simulink model "model_3"  (R2023b)
settings: Solver=VariableStepAuto  StartTime=0.0  StopTime=10  RelTol=1e-3
values from neighbouring files (symbols this model uses):
  k = acker(A, B, [s_b s_b s_b])    [obiekt.m]
settings Model: Creator=pavig  LastModifiedBy=pavig

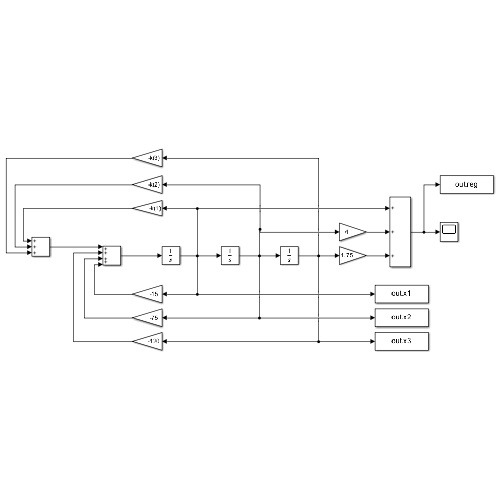
[thumbnail: Simulink's stored preview of the top-level diagram]
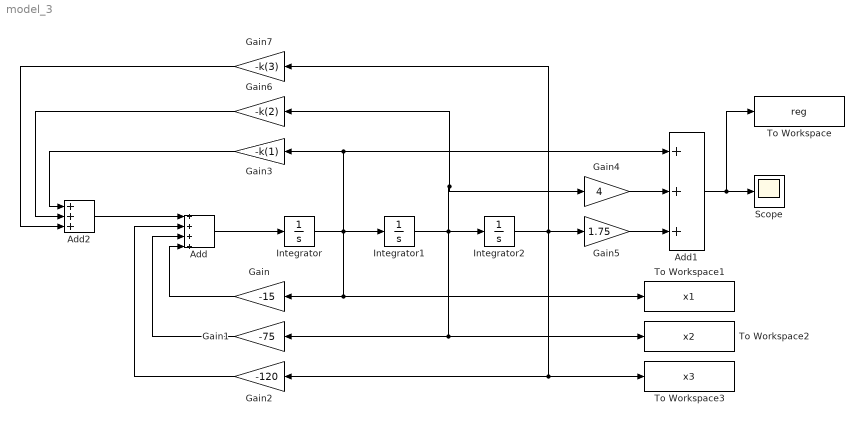
== system model_3 ==
  Add : Sum  Inputs=++++
  Add1 : Sum  Inputs=+++
  Add2 : Sum  Inputs=+++
  Gain : Gain  Gain=-15
  Gain1 : Gain  Gain=-75
  Gain2 : Gain  Gain=-120
  Gain3 : Gain  Gain=-k(1)
  Gain4 : Gain  Gain=4
  Gain5 : Gain  Gain=1.75
  Gain6 : Gain  Gain=-k(2)
  Gain7 : Gain  Gain=-k(3)
  Integrator : Integrator  InitialCondition=-1
  Integrator1 : Integrator  InitialCondition=2
  Integrator2 : Integrator  InitialCondition=1
  Scope : Scope
  To Workspace : ToWorkspace  VariableName=reg  SaveFormat=Timeseries  SampleTime=-1
  To Workspace1 : ToWorkspace  VariableName=x1  SaveFormat=Timeseries  SampleTime=-1
  To Workspace2 : ToWorkspace  VariableName=x2  SaveFormat=Timeseries  SampleTime=-1
  To Workspace3 : ToWorkspace  VariableName=x3  SaveFormat=Timeseries  SampleTime=-1
  wires:
  Integrator1/1 -> Gain6/1, Gain4/1, To Workspace2/1, Gain1/1, Integrator2/1
  Integrator/1 -> Gain3/1, Add1/1, To Workspace1/1, Gain/1, Integrator1/1
  Add1/1 -> To Workspace/1, Scope/1
  Integrator2/1 -> Gain7/1, Gain5/1, To Workspace3/1, Gain2/1
  Gain4/1 -> Add1/2
  Gain/1 -> Add/4
  Gain1/1 -> Add/3
  Gain5/1 -> Add1/3
  Add/1 -> Integrator/1
  Gain2/1 -> Add/2
  Add2/1 -> Add/1
  Gain3/1 -> Add2/1
  Gain6/1 -> Add2/2
  Gain7/1 -> Add2/3
